simulink model "pid_sys_id_model"  (R2024a)
settings: Solver=ode45  StartTime=0.0  StopTime=4  FixedStep=0.002  RelTol=1e-3  EnableMultiTasking=on
values from neighbouring files (symbols this model uses):
  Hm = H_high    [pid_sysID_stiffy.m]    (also in sysID_post.m = H_base * H_anti)
  Ts = 0.002    [sysID_init.m]    (also in sysID_stiffy.m)
libraries: quarc_library x2
settings Model: ExtModeTrigDuration=10000  Creator=quarc_user  LastModifiedBy=quarc_user
settings SolverCC: AlgebraicLoopSolver=TrustRegion  PositivePriorityOrder=on
settings DataIOCC: ReturnWorkspaceOutputs=off
settings DebuggingCC: UnconnectedInputMsg=warning  UnconnectedOutputMsg=warning  UnconnectedLineMsg=warning  ArithmeticOperatorsInVariantConditions=warning
settings ModelReferenceCC: EnableRefExpFcnMdlSchedulingChecks=on
settings SFSimCC: SimUseLocalCustomCode=off  CustomCodeUndefinedFunction=UseInterfaceOnly
settings RTWCC: Description=QUARC Win64 Target Using Toolchain  SystemTargetFile=quarc_win64.tlc  TemplateMakefile=quarc_default_tmf  RTWUseLocalCustomCode=off  Toolchain=QUARC win64 | nmake (64-bit Windows)  BuildConfiguration=Faster Runs  GPUComputeCapability=3.5
settings CodeAppCC: StateflowObjectComments=on
settings STFCustomTargetCC: ConcurrentExecutionCompliant=on  SystemTargetFile=quarc_win64.tlc
settings GRTTargetCC: ParMdlRefBuildCompliant=off  CompOptLevelCompliant=off  CombineOutputUpdateFcns=off  MatFileLogging=off  CPPClassGenCompliant=off  GRTInterface=on  ExtMode=on  ExtModeMexFile=quarc_comm
settings ConfigComp: CovMetricSettings=dswe

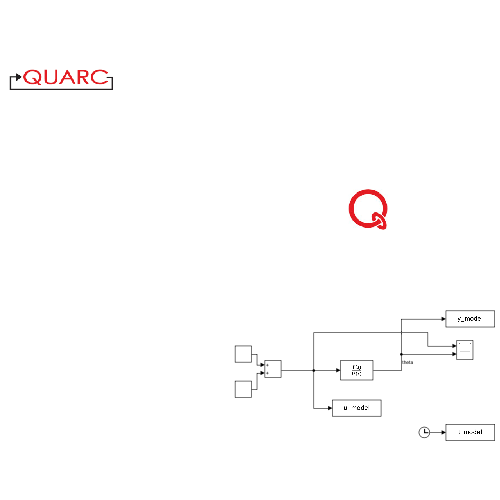
[thumbnail: Simulink's stored preview of the top-level diagram]
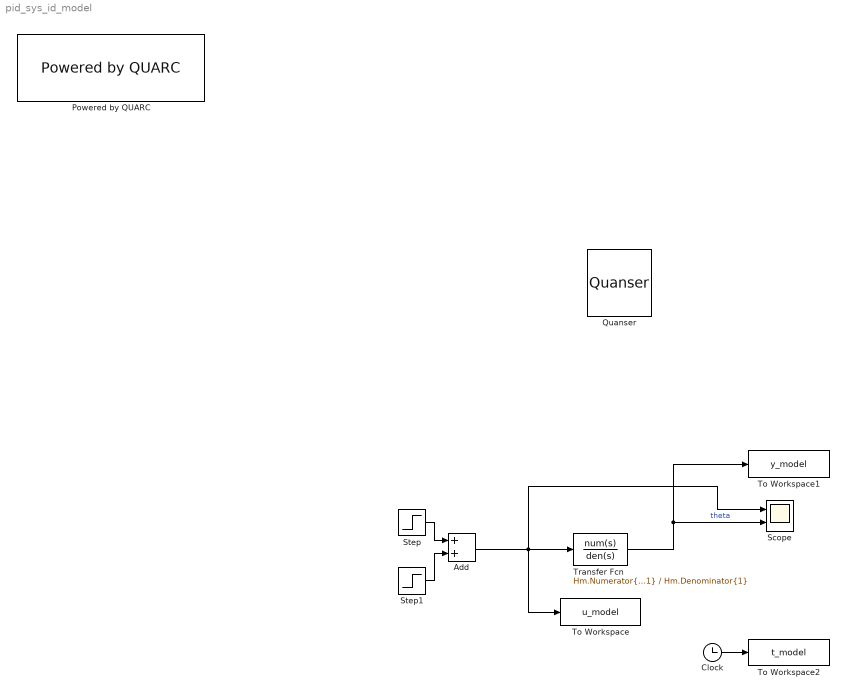
== system pid_sys_id_model ==
  Add : Sum
  Clock : Clock
  Powered by QUARC : quarc_library/Logos/Powered by QUARC
  Quanser : quarc_library/Logos/Quanser
  Scope : Scope  NumInputPorts=2
  Step : Step  Time=0  After=5  SampleTime=0
  Step1 : Step  Time=0.1  After=-5  SampleTime=0
  To Workspace : ToWorkspace  VariableName=u_model  SampleTime=Ts
  To Workspace1 : ToWorkspace  VariableName=y_model  SampleTime=Ts
  To Workspace2 : ToWorkspace  VariableName=t_model  SampleTime=Ts
  Transfer Fcn : TransferFcn  Numerator=Hm.Numerator{1}  Denominator=Hm.Denominator{1}
  wires:
  Step/1 -> Add/1
  Step1/1 -> Add/2
  Clock/1 -> To Workspace2/1
  Add/1 -> Transfer Fcn/1, Scope/1, To Workspace/1
  Transfer Fcn/1 -> To Workspace1/1, Scope/2  "theta"
